simulink model "MPCMGV"  (R2019a)
settings: Solver=FixedStepAuto  StartTime=0.0  StopTime=inf  FixedStep=0.005  RelTol=1e-3
InitFcn:
  | run('prepareSim')
libraries: delay x2
settings Model: Creator=wangz  LastModifiedBy=wangz
settings SolverCC: AlgebraicLoopSolver=LineSearch

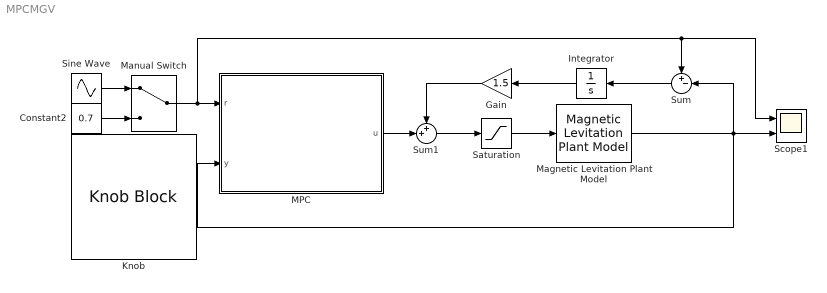
== system MPCMGV ==
  Constant2 : Constant  Value=0.7
  Gain : Gain  Gain=1.5
  Integrator : Integrator
  Knob : KnobBlock  ScaleMin=0.20000000000000001  ScaleMax=0.69999999999999996
  MPC : Subsystem
      mask Display: image('mask.png')
  Magnetic Levitation Plant Model : delay/Magnetic Levitation Plant Model  SystemSampleTime=-1
      mask Display: image('mask1.jpg')
  Manual Switch : ManualSwitch
  Saturation : Saturate  UpperLimit=1  LowerLimit=0
  Scope1 : Scope  NumInputPorts=2
  Sine Wave : Sin  Amplitude=0.25  Bias=0.4  Frequency=3  SampleTime=0
  Sum : Sum  Inputs=+-|
  Sum1 : Sum  Inputs=++|
  wires:
  Magnetic Levitation Plant Model/1 -> Sum/2, MPC/2("y "), Scope1/2
  MPC/1(u) -> Sum1/2
  Integrator/1 -> Gain/1
  Constant2/1 -> Manual Switch/2
  Manual Switch/1 -> Sum/1, Scope1/1, MPC/1("r ")
  Sine Wave/1 -> Manual Switch/1
  Saturation/1 -> Magnetic Levitation Plant Model/1
  Sum1/1 -> Saturation/1
  Sum/1 -> Integrator/1
  Gain/1 -> Sum1/1

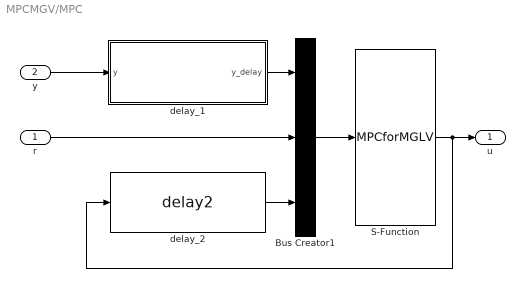
== system MPCMGV/MPC ==
  "r " : Inport
  "y " : Inport  Port=2
  Bus Creator1 : BusCreator  Inputs=3
  S-Function : S-Function  FunctionName=MPCforMGLV  Parameters=3,15  SFunctionDeploymentMode=off  EnableBusSupport=off
  delay_1 : Subsystem
  delay_2 : delay/delay2  SystemSampleTime=-1
  u : Outport
  wires:
  "r "/1 -> Bus Creator1/2
  Bus Creator1/1 -> S-Function/1
  "y "/1 -> delay_1/1("y ")
  delay_1/1(y_delay) -> Bus Creator1/1
  S-Function/1 -> delay_2/1, u/1
  delay_2/1 -> Bus Creator1/3

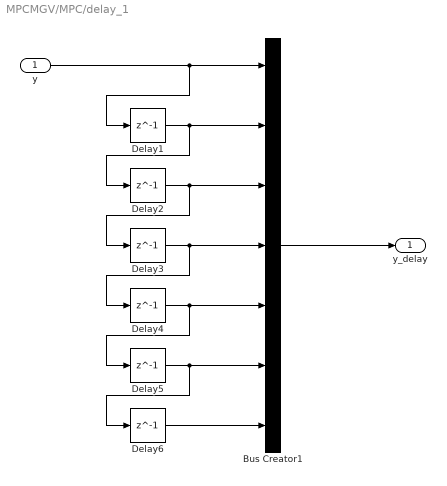
== system MPCMGV/MPC/delay_1 ==
  "y " : Inport
  Bus Creator1 : BusCreator  Inputs=7
  Delay{1..6} (6 alike) : Delay  DelayLength=1
  y_delay : Outport
  wires:
  "y "/1 -> Bus Creator1/1, Delay1/1
  Delay2/1 -> Bus Creator1/3, Delay3/1
  Delay5/1 -> Bus Creator1/6, Delay6/1
  Delay6/1 -> Bus Creator1/7
  Delay3/1 -> Bus Creator1/4, Delay4/1
  Delay4/1 -> Delay5/1, Bus Creator1/5
  Bus Creator1/1 -> y_delay/1
  Delay1/1 -> Delay2/1, Bus Creator1/2
